simulink model "uno"  (R2017a)
settings: Solver=VariableStepAuto  StartTime=0.0  StopTime=50  RelTol=1e-3
values from neighbouring files (symbols this model uses):
  a = 500    [uno.m]
  c = 400    [uno.m]
  F = 1000    [uno.m]
  M = 1000    [uno.m]
settings Model: Creator=Grażynka  LastModifiedBy=Grażynka

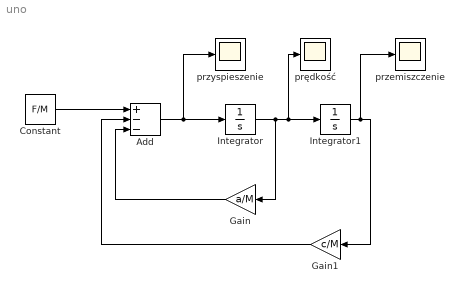
== system uno ==
  Add : Sum  Inputs=+--
  Constant : Constant  Value=F/M
  Gain : Gain  Gain=a/M
  Gain1 : Gain  Gain=c/M
  Integrator : Integrator
  Integrator1 : Integrator
  przemiszczenie : Scope
  przyspieszenie : Scope
  prędkość : Scope
  wires:
  Constant/1 -> Add/1
  Add/1 -> przyspieszenie/1, Integrator/1
  Integrator/1 -> Gain/1, prędkość/1, Integrator1/1
  Gain/1 -> Add/3
  Integrator1/1 -> przemiszczenie/1, Gain1/1
  Gain1/1 -> Add/2
